simulink model "dspwprfp"  (Simulink 6.0)
settings: Solver=FixedStepDiscrete  SolverMode=SingleTasking  StartTime=0.0  StopTime=1024  RelTol=1e-3
PreLoadFcn:
  | load dspwlets;
values from neighbouring files (symbols this model uses):
  hid = [-0.230377813309 0.714846570553 -0.63088076793 -0.027983769417 0.187034811719 0.030841381836 -0.032883011667 -0.010597401785]    [dspwlets.mat]
  hir = [-0.010597401785 -0.032883011667 0.030841381836 0.187034811719 -0.027983769417 -0.63088076793 0.714846570553 -0.230377813309]    [dspwlets.mat]
  lod = [-0.010597401785 0.032883011667 0.030841381836 -0.187034811719 -0.027983769417 0.63088076793 0.714846570553 0.230377813309]    [dspwlets.mat]
  lor = [0.230377813309 0.714846570553 0.63088076793 -0.027983769417 -0.187034811719 0.030841381836 0.032883011667 -0.010597401785]    [dspwlets.mat]
  ts = 1    [dspwlets.mat]    (also in lmsxy.m = [-1 0])
libraries: dspmlti4 x6, dspsigops x3, dspsrcs4 x1
settings Model: Creator=don  LastModifiedBy=schim  ExtModeTrigMode=oneshot  ExtModeArmWhenConnect=off
settings DataIOCC: LimitDataPoints=off  SaveOutput=off  SaveTime=off  SignalLoggingName=sigsOut
settings OptimizationCC: BlockReduction=off  BooleanDataType=off  MultiInstanced=off
settings FormatCC: IgnoreBidirectionalLines=off
settings DebuggingCC: IntegerOverflowMsg=none  ParameterPrecisionLossMsg=none
settings HardwareCC: TargetUnknown=on
settings CodeAppCC: SimulinkBlockComments=off
settings GRTTargetCC: TargetFcnLib=iso_c_tmw.mat

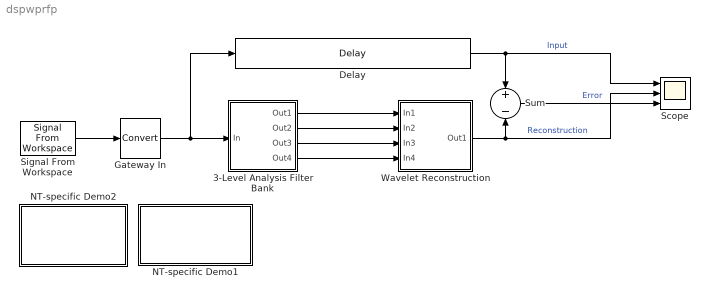
== system dspwprfp ==
  3-Level Analysis Filter Bank : Subsystem  mask{low=lod, high=hid}
      mask prompts: low "Lowpass FIR filter coefficients:"; high "Highpass FIR filter coefficients:"
  Delay : dspsigops/Delay  dly_unit=Samples  delay=7*(length(lod)-1)  ic_detail=on  dif_ic_for_ch=off  dif_ic_for_dly=off  ic=0  reset_popup=None
  Gateway In : DataTypeConversion  OutDataTypeMode=Specify via dialog  OutScaling=2^-10  RndMeth=Nearest  SaturateOnIntegerOverflow=on
  NT-specific Demo1 : Subsystem
      settings: OpenFcn=dspwprf
      mask Type: Frame-Based Demo
      mask Display: disp('Frame-Based\nDemo')
  NT-specific Demo2 : Subsystem
      settings: OpenFcn=dspwpr
      mask Type: Sample-Based Demo
      mask Display: disp('Sample-Based\nDemo')
  Scope : Scope  NumInputPorts=3
      settings: TimeRange=1200  YMin=-10~-10~-0.01  YMax=10~10~0.01
  Signal From Workspace : dspsrcs4/Signal From Workspace  X=noisdopp  Ts=ts  nsamps=1  OutputAfterFinalValue=Setting to zero
  Sum : Sum  Inputs=+-  SaturateOnIntegerOverflow=on  InputSameDT=on
  Wavelet Reconstruction : Subsystem
  wires:
  Signal From Workspace/1 -> Gateway In/1
  Wavelet Reconstruction/1(Out1) -> Sum/2, Scope/2  "Reconstruction"
  Sum/1 -> Scope/3  "Error"
  3-Level Analysis Filter Bank/1(Out1) -> Wavelet Reconstruction/1(In1)
  3-Level Analysis Filter Bank/2(Out2) -> Wavelet Reconstruction/2(In2)
  3-Level Analysis Filter Bank/3(Out3) -> Wavelet Reconstruction/3(In3)
  3-Level Analysis Filter Bank/4(Out4) -> Wavelet Reconstruction/4(In4)
  Delay/1 -> Scope/1, Sum/1  "Input"
  Gateway In/1 -> Delay/1, 3-Level Analysis Filter Bank/1(In)

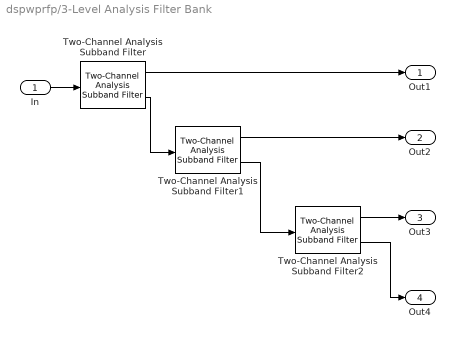
== system dspwprfp/3-Level Analysis Filter Bank ==
  In : Inport
  Two-Channel Analysis Subband Filter : dspmlti4/Two-Channel Analysis Subband Filter  DialogController=dspDDGCreate  DialogControllerArgs=DataTag0  lpf=low  hpf=high  framing=Maintain input frame size  accumMode=Binary point scaling  accumWordLength=32  accumFracLength=25  roundingMode=Nearest  overflowMode=on
      settings: allowOverrides=off
  Two-Channel Analysis Subband Filter1 : dspmlti4/Two-Channel Analysis Subband Filter  DialogController=dspDDGCreate  DialogControllerArgs=DataTag1  lpf=low  hpf=high  framing=Maintain input frame size  accumMode=Binary point scaling  accumWordLength=32  accumFracLength=25  roundingMode=Nearest  overflowMode=on
      settings: allowOverrides=off
  Two-Channel Analysis Subband Filter2 : dspmlti4/Two-Channel Analysis Subband Filter  DialogController=dspDDGCreate  DialogControllerArgs=DataTag2  lpf=low  hpf=high  framing=Maintain input frame size  accumMode=Binary point scaling  accumWordLength=32  accumFracLength=25  roundingMode=Nearest  overflowMode=on
      settings: allowOverrides=off
  Out1 : Outport
  Out2 : Outport  Port=2
  Out3 : Outport  Port=3
  Out4 : Outport  Port=4
  wires:
  In/1 -> Two-Channel Analysis Subband Filter/1
  Two-Channel Analysis Subband Filter/1 -> Out1/1
  Two-Channel Analysis Subband Filter/2 -> Two-Channel Analysis Subband Filter1/1
  Two-Channel Analysis Subband Filter1/1 -> Out2/1
  Two-Channel Analysis Subband Filter2/1 -> Out3/1
  Two-Channel Analysis Subband Filter2/2 -> Out4/1
  Two-Channel Analysis Subband Filter1/2 -> Two-Channel Analysis Subband Filter2/1

== system dspwprfp/NT-specific Demo1 ==

== system dspwprfp/NT-specific Demo2 ==

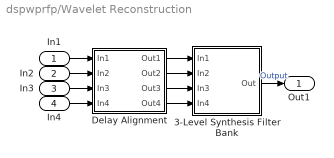
== system dspwprfp/Wavelet Reconstruction ==
  In1 : Inport
  In2 : Inport  Port=2
  In3 : Inport  Port=3
  In4 : Inport  Port=4
  3-Level Synthesis Filter Bank : Subsystem  mask{low=lor, high=hir}
      mask prompts: low "Lowpass FIR filter coefficients:"; high "Highpass FIR filter coefficients:"
  Delay Alignment : Subsystem
  Out1 : Outport
  wires:
  In4/1 -> Delay Alignment/4(In4)
  In3/1 -> Delay Alignment/3(In3)
  3-Level Synthesis Filter Bank/1(Out) -> Out1/1  "Output"
  In2/1 -> Delay Alignment/2(In2)
  In1/1 -> Delay Alignment/1(In1)
  Delay Alignment/4(Out4) -> 3-Level Synthesis Filter Bank/4(In4)
  Delay Alignment/3(Out3) -> 3-Level Synthesis Filter Bank/3(In3)
  Delay Alignment/2(Out2) -> 3-Level Synthesis Filter Bank/2(In2)
  Delay Alignment/1(Out1) -> 3-Level Synthesis Filter Bank/1(In1)

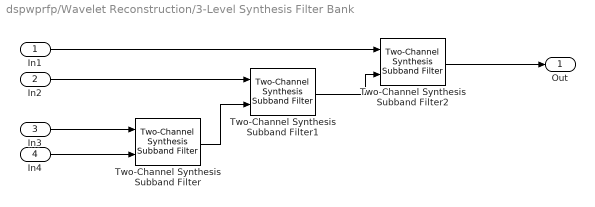
== system dspwprfp/Wavelet Reconstruction/3-Level Synthesis Filter Bank ==
  In1 : Inport
  In2 : Inport  Port=2
  In3 : Inport  Port=3
  In4 : Inport  Port=4
  Two-Channel Synthesis Subband Filter : dspmlti4/Two-Channel Synthesis Subband Filter  DialogController=dspDDGCreate  DialogControllerArgs=DataTag3  lpf=low  hpf=high  framing=Maintain input frame size  accumMode=Binary point scaling  accumWordLength=32  accumFracLength=25  roundingMode=Nearest  overflowMode=on
      settings: allowOverrides=off
  Two-Channel Synthesis Subband Filter1 : dspmlti4/Two-Channel Synthesis Subband Filter  DialogController=dspDDGCreate  DialogControllerArgs=DataTag4  lpf=low  hpf=high  framing=Maintain input frame size  accumMode=Binary point scaling  accumWordLength=32  accumFracLength=25  roundingMode=Nearest  overflowMode=on
      settings: allowOverrides=off
  Two-Channel Synthesis Subband Filter2 : dspmlti4/Two-Channel Synthesis Subband Filter  DialogController=dspDDGCreate  DialogControllerArgs=DataTag5  lpf=low  hpf=high  framing=Maintain input frame size  accumMode=Binary point scaling  accumWordLength=32  accumFracLength=25  roundingMode=Nearest  overflowMode=on
      settings: allowOverrides=off
  Out : Outport
  wires:
  In3/1 -> Two-Channel Synthesis Subband Filter/1
  In4/1 -> Two-Channel Synthesis Subband Filter/2
  In2/1 -> Two-Channel Synthesis Subband Filter1/1
  Two-Channel Synthesis Subband Filter/1 -> Two-Channel Synthesis Subband Filter1/2
  In1/1 -> Two-Channel Synthesis Subband Filter2/1
  Two-Channel Synthesis Subband Filter1/1 -> Two-Channel Synthesis Subband Filter2/2
  Two-Channel Synthesis Subband Filter2/1 -> Out/1

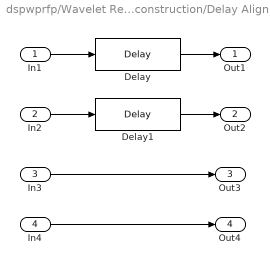
== system dspwprfp/Wavelet Reconstruction/Delay Alignment ==
  In1 : Inport
  In2 : Inport  Port=2
  In3 : Inport  Port=3
  In4 : Inport  Port=4
  Delay : dspsigops/Delay  dly_unit=Samples  delay=3*(length(lod)-1)  ic_detail=off  dif_ic_for_ch=off  dif_ic_for_dly=off  ic=0  reset_popup=None
  Delay1 : dspsigops/Delay  dly_unit=Samples  delay=length(lod) - 1  ic_detail=off  dif_ic_for_ch=off  dif_ic_for_dly=off  ic=0  reset_popup=None
  Out1 : Outport
  Out2 : Outport  Port=2
  Out3 : Outport  Port=3
  Out4 : Outport  Port=4
  wires:
  Delay/1 -> Out1/1
  In1/1 -> Delay/1
  Delay1/1 -> Out2/1
  In2/1 -> Delay1/1
  In4/1 -> Out4/1
  In3/1 -> Out3/1
